simulink model "PumpModels_quadraticCharacter"  (R2018b)
settings: Solver=VariableStepAuto  StartTime=0.0  StopTime=10.0  RelTol=1e-3
undefined symbols (not defined in the file): DiameterLastPiece, DPConstant, DPLinear, DPQuadratic, ID, MassFlow, path_carnot, Pressure, Temperature, Water
libraries: carnot x7
settings Model: Creator=drhf  LastModifiedBy=drhf

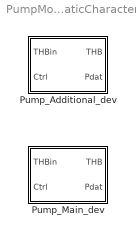
== system PumpModels_quadraticCharacter ==
  Pump_Additional_dev : Subsystem  mask(Pump Additional){Tini=20, PathName=fullfile(path_carnot('libsl'), 'Hydraulics', 'Pump_Main', 'parameter_set'), FileName='Pump5m.mat', userPath=off, userParam=off, a0=50000, a1=-45000, a2=0, dia=0.025, UA=1, mcp=4182, e0=35, e1=22.5, e2=-8.1}
      mask prompts: Tini "Ambient temperature for losses and initial temperture in °C"; PathName "Path"; FileName "Parameter set"; userPath "Edit path and name of parameter set"; userParam "User defined parameters"; a0 "a0: pump head in [Pa] (pressure increase at zero flow)"; a1 "a1: pump characteristic linear coefficient [Pa*s/kg]"; a2 "a2: pump characteristic quadratic coefficient [Pa*(s/kg)²]"; dia "Diameter at in- and outlet [m]"; UA "UA: thermal loss coefficient in W/K"; mcp "mcp: thermal capacity of the node in J/K"; e0 "e0: constant coefficient in W"; e1 "e1: linear coefficient in W*s/kg"; e2 "e2: quadratic coefficient in W*(s/kg)²"
      mask help:
      | This is an additional pump in a circuit. Every circuit must have exactly ONE 'Pump_Main'. It may have several 'Pump_Additional' blocks. The pump adds pump_head to the pressure drop of the circuit dp_circuit:
      |     dp_circuit = c + l*mdot + q*(mdot)²
      |     pump_head_ = a0*Ctrl² + a1*Ctrl*mdot +a2*mdot²
      |     dp_total = pump_head - dp_circuit
      |     p1 = system_pressure + (a0*Ctrl² - c) + (a1*Ctrl - l) * mdot + (a2-q)*(mdot)²
      | with
      |   Ctrl : Control signal input [0..1]
      | Note: Pump_Additional uses the parameters sets as Pump_Main.
      mask init:
      | % callback to set parameters of model
      | [ok, param] = CarnotCallbacks_PumpAdditional('SetParameters',gcbh,PathName,FileName);
      mask Help: web(fullfile(path_carnot('help'),'Pump_Main.html'),'-helpbrowser')
      mask TypeOptions Tini: ThermalNodeTHB/Tini
      mask Callback userPath: [ok, param] = CarnotCallbacks_PumpAdditional('UserEdit',gcbh);
      mask Callback userParam: [ok, param] = CarnotCallbacks_PumpAdditional('UserEdit',gcbh);
      mask TypeOptions a0: PumpHead/Gain
      mask TypeOptions a1: PumpLinear/Gain
      mask TypeOptions a2: PumpQuadratic/Value
      mask TypeOptions dia: dia/Value
      mask TypeOptions UA: ThermalNodeTHB/UA
      mask TypeOptions mcp: ThermalNodeTHB/mcp
      mask TypeOptions e0: ElectricConsumptionPump/e0
      mask TypeOptions e1: ElectricConsumptionPump/e1
      mask TypeOptions e2: ElectricConsumptionPump/e2
      mask DialogControl ParameterGroupFile Prompt: Picking a parameter set
      mask DialogControl Control1 Prompt: Carnot public data
      mask DialogControl Control1 Callback: [ok, file] = CarnotCallbacks_PumpAdditional('GetFilename',gcbh,'public');
      mask DialogControl Control3 Prompt: Carnot internal data
      mask DialogControl Control3 Callback: [ok, file] = CarnotCallbacks_PumpAdditional('GetFilename',gcbh,'internal');
      mask DialogControl Control4 Prompt: Selected path
      mask DialogControl Control4 Callback: [ok, file] = CarnotCallbacks_PumpAdditional('GetFilename',gcbh,'selected');
      mask DialogControl PrameterGroupUser Prompt: Parameter Values
      mask DialogControl Container9 Prompt: Hydraulic
      mask DialogControl Container7 Prompt: Thermal
      mask DialogControl Control9 Prompt: Thermal node for temperature:  mcp * dTnode/dt = UA*(Tamb-Tnode) + mdot*cp_in*(Tin-Tnode)
      mask DialogControl Container12 Prompt: Electric
      mask DialogControl Control7 Prompt: Power consumption  Pel = e0 + e1*mdot + e2*mdot²
      mask DialogControl Control5 Prompt: Save in Carnot internal data
      mask DialogControl Control5 Callback: [ok, param] = CarnotCallbacks_PumpAdditional('SaveFilename',gcbh,'internal','B');
      mask DialogControl Control6 Prompt: Save in selected path
      mask DialogControl Control6 Callback: [ok, param] = CarnotCallbacks_PumpAdditional('SaveFilename',gcbh,'selected','B');
      mask Display:
      | % user defined picture file
      | picfile = fullfile(path_carnot('intlibsl'), ...
      |         'Hydraulics', 'Pump_Additional', 'PumpAdditional.jpg');
      | 
      | pic = false;
      | if ~BlockIsInCarnotLibrary    % if not located in library any more
      |     if exist(picfile,'file') % show internal picture if defined
      |         image(imread(picfile), [0.2, 0, 0.6, 1])
      |         set_param(gcb, 'BackgroundColor', 'White')
      |         pic = true;
      |     end
      | end
      | if ~pic    % show public picture
      |     set_param(gcb, 'BackgroundColor', 'green')
      |     plot(0,0,1,1,[40,70,40,30,30,40,60,70,70,60,40]/100, ...
      |         [70,50,30,40,60,70,70,60,40,30,30]/100)
      |     disp('add')
      | end
  Pump_Main_dev : Subsystem  mask(Pump Main){Tini=20, p0=3e5, IDpreset=pressure drop, fluid=Water, mix=0, mix2=0, mix3=0, t1=0.1, PathName=fullfile(path_carnot('libsl'), 'Hydraulics', 'Pump_Main', 'parameter_set'), FileName='Pump6m.mat', userPath=off, userParam=off, a0=60000, a1=-43200, a2=0, dia=0.025, UA=1, mcp=4182, e0=50, e1=28.8, e2=-10.368}
      mask prompts: Tini "Ambient temperature for losses and initial temperture in °C"; p0 "System pressure at pump inlet [Pa]"; IDpreset "Pressure calculation"; mix "Fluid mixture    [0..1]"; mix2 "Fluid mixture 2 [0..1]"; mix3 "Fluid mixture 3 [0..1]"; t1 "Time constant [s] of PT1 transfer function for massflow"; PathName "Path"; FileName "Parameter set"; userPath "Edit path and name of parameter set"; userParam "User defined parameters"; a0 "a0: pump head in [Pa] (pressure increase at zero flow)"; a1 "a1: pump characteristic linear coefficient [Pa*s/kg]"; a2 "a2: pump characteristic quadratic coefficient [Pa*(s/kg)²]"; dia "Diameter at in- and outlet [m]"; UA "UA: thermal loss coefficient in W/K"; mcp "mcp: thermal capacity of the node in J/K"; e0 "e0: constant coefficient in W"; e1 "e1: linear coefficient in W*s/kg"; e2 "e2: quadratic coefficient in W*(s/kg)²"
      mask help:
      | This is the main pump in a circuit. Every circuit must have exactly ONE 'Pump_Main'. Use the 'Pump_Additional' blocks if you want to use more pumps.
      | The Pump_Main calculate massflow by setting pressure drop in the circuit (dp_circuit) equal to the pressure increase of the pump (pump_head).
      |   dp_circuit = c + l*mdot + q*mdot²
      |   pump_head_ = a0*Ctrl² + a1*Ctrl*mdot +a2*mdot²
      | with
      |   mdot : massflow in kg/s
      |   Ctrl : Control signal input [0..1]
      mask init:
      | % callback to set parameters of model
      | [ok, param] = CarnotCallbacks_PumpMain('SetParameters',gcbh,PathName,FileName);
      mask Help: web(fullfile(path_carnot('help'),'Pump_Main.html'),'-helpbrowser')
      mask TypeOptions Tini: ThermalNodeTHB/Tini
      mask TypeOptions p0: basic_THB/p
      mask TypeOptions IDpreset: ID/IDpreset
      mask TypeOptions fluid: basic_THB/fluid
      mask TypeOptions mix: basic_THB/mix
      mask TypeOptions mix2: basic_THB/mix2
      mask TypeOptions mix3: basic_THB/mix3
      mask TypeOptions t1: Transfer Fcn/t1
      mask Callback userPath: [ok, param] = CarnotCallbacks_PumpMain('UserEdit',gcbh);
      mask Callback userParam: [ok, param] = CarnotCallbacks_PumpMain('UserEdit',gcbh);
      mask TypeOptions a0: PumpHead/Gain
      mask TypeOptions a1: PumpLinear/Value
      mask TypeOptions a2: PumpQuadratic/Value
      mask TypeOptions dia: basic_THB/dia
      mask TypeOptions UA: ThermalNodeTHB/UA
      mask TypeOptions mcp: ThermalNodeTHB/mcp
      mask TypeOptions e0: ElectricConsumptionPump/e0
      mask TypeOptions e1: ElectricConsumptionPump/e1
      mask TypeOptions e2: ElectricConsumptionPump/e2
      mask DialogControl ParameterGroupFile Prompt: Picking a parameter set
      mask DialogControl Control1 Prompt: Carnot public data
      mask DialogControl Control1 Callback: [ok, file] = CarnotCallbacks_PumpMain('GetFilename',gcbh,'public');
      mask DialogControl Control3 Prompt: Carnot internal data
      mask DialogControl Control3 Callback: [ok, file] = CarnotCallbacks_PumpMain('GetFilename',gcbh,'internal');
      mask DialogControl Control4 Prompt: Selected path
      mask DialogControl Control4 Callback: [ok, file] = CarnotCallbacks_PumpMain('GetFilename',gcbh,'selected');
      mask DialogControl PrameterGroupUser Prompt: Parameter Values
      mask DialogControl Container9 Prompt: Hydraulic
      mask DialogControl Container7 Prompt: Thermal
      mask DialogControl Control9 Prompt: Thermal node for temperature:  mcp * dTnode/dt = UA*(Tamb-Tnode) + mdot*cp_in*(Tin-Tnode)
      mask DialogControl Container14 Prompt: Electric
      mask DialogControl Control7 Prompt: Power consumption  Pel = e0 + e1*mdot + e2*mdot²
      mask DialogControl Control5 Prompt: Save in Carnot internal data
      mask DialogControl Control5 Callback: [ok, param] = CarnotCallbacks_PumpMain('SaveFilename',gcbh,'internal','B');
      mask DialogControl Control6 Prompt: Save in selected path
      mask DialogControl Control6 Callback: [ok, param] = CarnotCallbacks_PumpMain('SaveFilename',gcbh,'selected','B');
      mask Display:
      | % user defined picture file
      | picfile = fullfile(path_carnot('intlibsl'), ...
      |         'Hydraulics', 'Pump_Main', 'PumpMain.jpg');
      | 
      | pic = false;
      | if ~BlockIsInCarnotLibrary    % if not located in library any more
      |     if exist(picfile,'file') % show internal picture if defined
      |         image(imread(picfile), [0.2, 0, 0.6, 1])
      |         set_param(gcb, 'BackgroundColor', 'White')
      |         pic = true;
      |     end
      | end
      | if ~pic    % show public picture
      |     set_param(gcb, 'BackgroundColor', 'green')
      |     plot(0,0,1,1,[40,70,40,30,30,40,60,70,70,60,40]/100, ...
      |         [70,50,30,40,60,70,70,60,40,30,30]/100)
      |     disp('main')
      | end

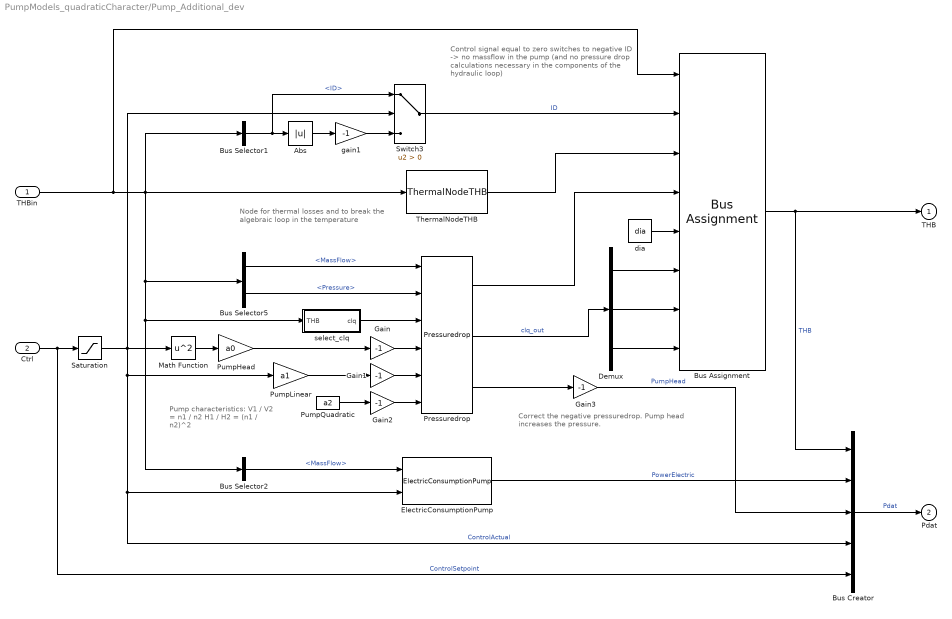
== system PumpModels_quadraticCharacter/Pump_Additional_dev ==
  note: Pump characteristics:
      | V1 / V2 = n1 / n2
      | H1 / H2 = (n1 / n2)^2
  note: Correct the negative pressuredrop.
      | Pump head increases the pressure.
  note: Control signal equal to zero switches
      | to negative ID -> no massflow in the
      | pump (and no pressure drop calculations
      | necessary in the components of the
      | hydraulic loop)
  note: Node for thermal losses and to break
      | the algebraic loop in the temperature
  THBin : Inport
  Ctrl : Inport  Port=2
  Abs : Abs
  Bus Assignment : BusAssignment  AssignedSignals=ID,Temperature,Pressure,DiameterLastPiece,DPConstant,DPLinear,DPQuadratic
  Bus Creator : BusCreator  Inputs=5
  Bus Selector1 : BusSelector  OutputSignals=ID
  Bus Selector2 : BusSelector  OutputSignals=MassFlow
  Bus Selector5 : BusSelector  OutputSignals=MassFlow,Pressure
  Demux : Demux  Outputs=3
  ElectricConsumptionPump : carnot/Basic/Hydraulics/ElectricConsumptionPump  e0=e0  e1=e1  e2=e2
  Gain{,1..3} (4 alike) : Gain  Gain=-1
  Math Function : Math  Operator=square  SaturateOnIntegerOverflow=on
  Pressuredrop : carnot/Basic/Pressure_Drop/Pressuredrop
  PumpHead : Gain  Gain=a0
  PumpLinear : Gain  Gain=a1
  PumpQuadratic : Constant  Value=a2
  Saturation : Saturate  UpperLimit=1  LowerLimit=0
  Switch3 : Switch  Criteria=u2 > Threshold  SaturateOnIntegerOverflow=on  InputSameDT=on
  ThermalNodeTHB : carnot/Basic/Thermal_Models/ThermalNodeTHB  UA=UA  mcp=mcp  Tini=Tini
  dia : Constant  Value=dia
  gain1 : Gain  Gain=-1  SaturateOnIntegerOverflow=on  OutDataTypeStr=Inherit: Same as input  ParamDataTypeStr=Inherit: Same as input
  select_clq : Subsystem
  THB : Outport
  Pdat : Outport  Port=2
  wires:
  Math Function/1 -> PumpHead/1
  Saturation/1 -> Switch3/2, PumpLinear/1, Bus Creator/4, ElectricConsumptionPump/2, Math Function/1  "ControlActual"
  Gain3/1 -> Bus Creator/3  "PumpHead"
  Pressuredrop/1 -> Bus Assignment/4
  Pressuredrop/2 -> Demux/1  "clq_out"
  Pressuredrop/3 -> Gain3/1
  Bus Assignment/1 -> THB/1, Bus Creator/1  "THB"
  Bus Selector2/1 -> ElectricConsumptionPump/1  "<MassFlow>"
  Bus Creator/1 -> Pdat/1  "Pdat"
  ElectricConsumptionPump/1 -> Bus Creator/2  "PowerElectric"
  Ctrl/1 -> Saturation/1, Bus Creator/5  "ControlSetpoint"
  Bus Selector1/1 -> Switch3/1, Abs/1  "<ID>"
  Abs/1 -> gain1/1
  gain1/1 -> Switch3/3
  Switch3/1 -> Bus Assignment/2  "ID"
  Bus Selector5/1 -> Pressuredrop/1  "<MassFlow>"
  dia/1 -> Bus Assignment/5
  THBin/1 -> Bus Selector1/1, Bus Selector2/1, select_clq/1(THB), Bus Selector5/1, ThermalNodeTHB/1, Bus Assignment/1
  PumpHead/1 -> Gain/1
  PumpLinear/1 -> Gain1/1
  PumpQuadratic/1 -> Gain2/1
  Demux/1 -> Bus Assignment/6
  Demux/2 -> Bus Assignment/7
  Demux/3 -> Bus Assignment/8
  ThermalNodeTHB/1 -> Bus Assignment/3
  select_clq/1(clq) -> Pressuredrop/3
  Bus Selector5/2 -> Pressuredrop/2  "<Pressure>"
  Gain/1 -> Pressuredrop/4
  Gain1/1 -> Pressuredrop/5
  Gain2/1 -> Pressuredrop/6

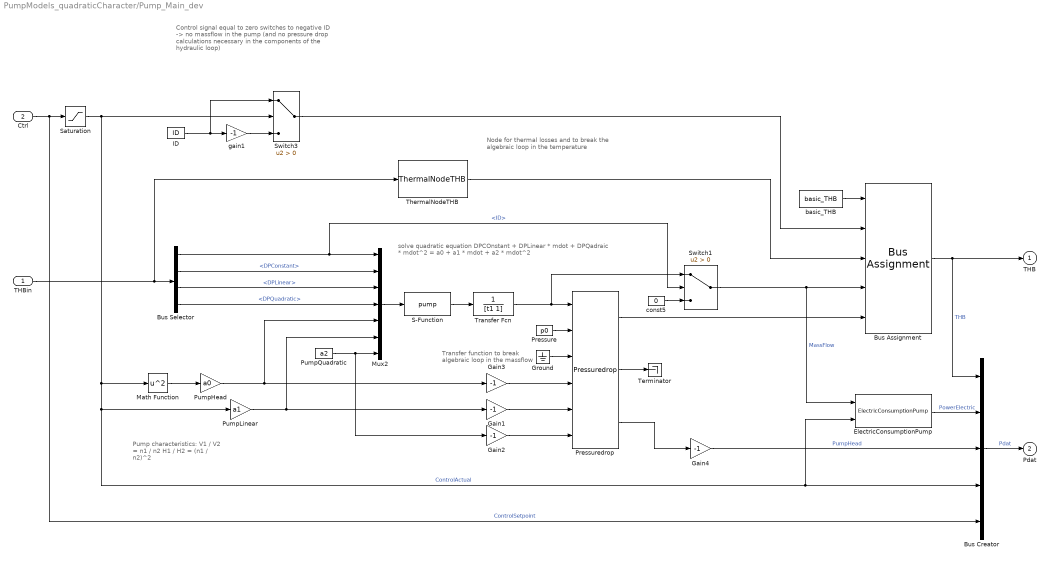
== system PumpModels_quadraticCharacter/Pump_Main_dev ==
  note: Pump characteristics:
      | V1 / V2 = n1 / n2
      | H1 / H2 = (n1 / n2)^2
  note: Control signal equal to zero switches
      | to negative ID -> no massflow in the
      | pump (and no pressure drop calculations
      | necessary in the components of the
      | hydraulic loop)
  note: solve quadratic equation
      | DPCOnstant + DPLinear * mdot + DPQadraic * mdot^2
      | = a0 + a1 * mdot + a2 * mdot^2
  note: Transfer function to
      | break algebraic loop
      | in the massflow
  note: Node for thermal losses and to break
      | the algebraic loop in the temperature
  THBin : Inport
  Ctrl : Inport  Port=2
  Bus Assignment : BusAssignment  AssignedSignals=ID,Temperature,MassFlow,Pressure
  Bus Creator : BusCreator  Inputs=5
  Bus Selector : BusSelector  OutputSignals=ID,DPConstant,DPLinear,DPQuadratic
  ElectricConsumptionPump : carnot/Basic/Hydraulics/ElectricConsumptionPump  e0=e0  e1=e1  e2=e2
  Gain{1..4} (4 alike) : Gain  Gain=-1
  Ground : Ground
  ID : Constant  Value=ID  mask{IDpreset=pressure drop}
      mask prompts: IDpreset "Calculation"
      mask init:
      | ID = IDpreset*10000 + 1;
      mask TypeOptions IDpreset: pressure drop | pressure drop and pressure head
  Math Function : Math  Operator=square  SaturateOnIntegerOverflow=on
  Mux2 : Mux  Inputs=7
  Pressure : Constant  Value=p0
  Pressuredrop : carnot/Basic/Pressure_Drop/Pressuredrop
  PumpHead : Gain  Gain=a0
  PumpLinear : Gain  Gain=a1
  PumpQuadratic : Constant  Value=a2
  S-Function : S-Function  FunctionName=pump  SFunctionDeploymentMode=off  EnableBusSupport=off
  Saturation : Saturate  UpperLimit=1  LowerLimit=0
  Switch1 : Switch  Criteria=u2 > Threshold  SaturateOnIntegerOverflow=on  InputSameDT=on
  Switch3 : Switch  Criteria=u2 > Threshold  SaturateOnIntegerOverflow=on  InputSameDT=on
  Terminator : Terminator
  ThermalNodeTHB : carnot/Basic/Thermal_Models/ThermalNodeTHB  UA=UA  mcp=mcp  Tini=Tini
  Transfer Fcn : TransferFcn  Denominator=[t1 1]  mask{t1=t1}
      mask prompts: t1 "Time constant of PT1 transfer function for massflow in s"
  basic_THB : carnot/Basic/Hydraulics/basic_THB  t=20  mdot=0  p=p0  ID=No Pressure Drop  fluid=Water  mix=mix  mix2=mix2  mix3=mix3  dia=dia  hgt=0
  const5 : Constant  Value=0
  gain1 : Gain  Gain=-1  SaturateOnIntegerOverflow=on  OutDataTypeStr=Inherit: Same as input  ParamDataTypeStr=Inherit: Same as input
  THB : Outport
  Pdat : Outport  Port=2
  wires:
  Math Function/1 -> PumpHead/1
  Gain4/1 -> Bus Creator/3  "PumpHead"
  Gain2/1 -> Pressuredrop/6
  Gain1/1 -> Pressuredrop/5
  Gain3/1 -> Pressuredrop/4
  Saturation/1 -> Bus Creator/4, ElectricConsumptionPump/2, PumpLinear/1, Math Function/1, Switch3/2  "ControlActual"
  Pressuredrop/2 -> Terminator/1
  Ground/1 -> Pressuredrop/3
  Pressuredrop/1 -> Bus Assignment/5
  Pressure/1 -> Pressuredrop/2
  Bus Selector/4 -> Mux2/4  "<DPQuadratic>"
  Bus Selector/3 -> Mux2/3  "<DPLinear>"
  Bus Selector/2 -> Mux2/2  "<DPConstant>"
  ThermalNodeTHB/1 -> Bus Assignment/3
  Switch3/1 -> Bus Assignment/2
  Bus Assignment/1 -> Bus Creator/1, THB/1  "THB"
  basic_THB/1 -> Bus Assignment/1
  const5/1 -> Switch1/3
  Transfer Fcn/1 -> Switch1/1, Pressuredrop/1
  gain1/1 -> Switch3/3
  ID/1 -> gain1/1, Switch3/1
  Ctrl/1 -> Bus Creator/5, Saturation/1  "ControlSetpoint"
  PumpHead/1 -> Gain3/1, Mux2/5
  PumpQuadratic/1 -> Gain2/1, Mux2/7
  PumpLinear/1 -> Mux2/6, Gain1/1
  S-Function/1 -> Transfer Fcn/1
  Mux2/1 -> S-Function/1
  Switch1/1 -> ElectricConsumptionPump/1, Bus Assignment/4  "MassFlow"
  Bus Selector/1 -> Mux2/1, Switch1/2  "<ID>"
  Pressuredrop/3 -> Gain4/1
  THBin/1 -> ThermalNodeTHB/1, Bus Selector/1
  Bus Creator/1 -> Pdat/1  "Pdat"
  ElectricConsumptionPump/1 -> Bus Creator/2  "PowerElectric"

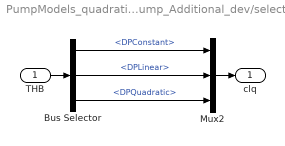
== system PumpModels_quadraticCharacter/Pump_Additional_dev/select_clq ==
  THB : Inport
  Bus Selector : BusSelector  OutputSignals=DPConstant,DPLinear,DPQuadratic
  Mux2 : Mux  Inputs=3
  clq : Outport
  wires:
  Mux2/1 -> clq/1
  THB/1 -> Bus Selector/1
  Bus Selector/1 -> Mux2/1  "<DPConstant>"
  Bus Selector/2 -> Mux2/2  "<DPLinear>"
  Bus Selector/3 -> Mux2/3  "<DPQuadratic>"
